simulink model "lab4"  (Simulink 8.5)
settings: Solver=ode45  StartTime=0.0  StopTime=10000  RelTol=1e-3
settings Model: Creator=Kirill  LastModifiedBy=Meteo
settings DebuggingCC: SolverPrmCheckMsg=warning  FcnCallInpInsideContextMsg=UseLocalSettings
settings SimEventsCC: propDiagAttribOutput=1  propDiagFcnCallOutput=1  propDiagStatOutput=0  propPreventDuplicateEvents=0

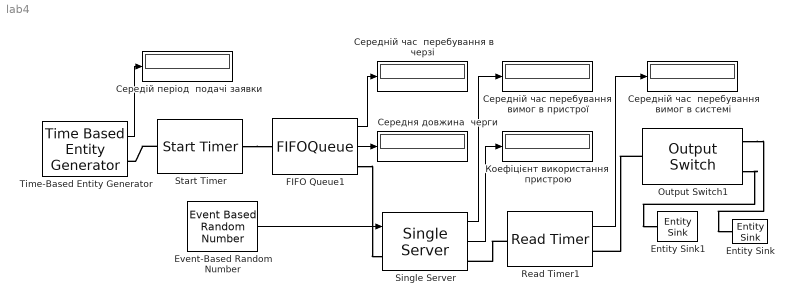
== system lab4 ==
  "Entity Sink " : EntitySink
  Entity Sink1 : EntitySink
  Event-Based Random Number : EventBasedRandomNumber  meanExp=17
  FIFO Queue1 : FIFOQueue  StatAverageWait=on  StatAverageQueueLength=on
      settings: OutputPortMap=o2,o3
  Output Switch1 : OutputSwitch  NumberOutputPorts=2
  Read Timer1 : ReadTimer  StatAverageTimeElapsed=on
      settings: OutputPortMap=o3
  Single Server : SingleServer  ServiceTimeFrom=Signal port t  StatAverageWait=on  StatUtilization=on
      settings: OutputPortMap=o4,o5
  Start Timer : StartTimer
  Time-Based Entity Generator : TimeBasedEntityGenerator  Distribution=Exponential  Period=27  Mean=27  PriorityEntityGeneration=2000  StatAverageIntergenerationTime=on
      settings: OutputPortMap=o2
  Коефіцієнт використання  пристрою : Display
  Середня довжина  черги : Display
  Середній час  перебування в черзі : Display
  Середній час  перебування вимог в системі : Display
  "Середній час перебування  вимог в пристрої " : Display
  Середій період  подачі заявки : Display
  wires:
  FIFO Queue1/1 -> Середній час  перебування в черзі/1
  Single Server/1 -> "Середній час перебування  вимог в пристрої "/1
  Read Timer1/1 -> Середній час  перебування вимог в системі/1
  Single Server/2 -> Коефіцієнт використання  пристрою/1
  FIFO Queue1/2 -> Середня довжина  черги/1
  Event-Based Random Number/1 -> Single Server/1
  Time-Based Entity Generator/1 -> Середій період  подачі заявки/1
  connections:
  Start Timer/LConn1 -- Time-Based Entity Generator/RConn1
  Start Timer/RConn1 -- FIFO Queue1/LConn1
  FIFO Queue1/RConn1 -- Single Server/LConn1
  Read Timer1/LConn1 -- Single Server/RConn1
  Output Switch1/LConn1 -- Read Timer1/RConn1
  Output Switch1/RConn1 -- "Entity Sink "/LConn1
  Output Switch1/RConn2 -- Entity Sink1/LConn1
